simulink model "ep_DDMR_5Methods"  (Simulink 5.0)
settings: Solver=ode45  StartTime=0.0  StopTime=15  MaxStep=.1  MinStep=.001  RelTol=1e-3
values from neighbouring files (symbols this model uses):
  Gc = [2 2 3 4]    [init_ddmr.m]
  I_status = 0    [init_ddmr.m]
  IL_status = 1    [init_ddmr.m]
  PDIL_status = [1 2]    [init_ddmr.m]
libraries: dspsigattribs x15, dspmtrx3 x13, simulink x11, dspinverses x1
settings Model: LastModifiedBy=begawan  InitialStep=.001  MaxDataPoints=10000  BooleanDataType=off

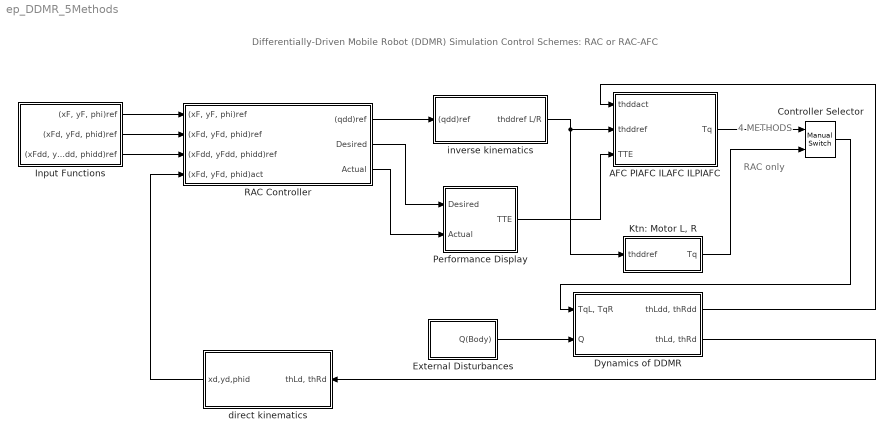
== system ep_DDMR_5Methods ==
  note: Differentially-Driven Mobile Robot (DDMR) Simulation
      | Control Schemes: RAC or RAC-AFC
  note: 4 METHODS
  note: RAC only
  "AFC PIAFC ILAFC ILPIAFC " : Subsystem  mask(6){GcAFC=on, GcPIAFC=off, GcILAFC=off, GcILPIAFC=off, pureIN=[2.4;2.4], PPhai=[0.2;0.2], DLa=[0.1;0.1], IN=[2.675;2.675], DIN=[0.71;0.71], Phai=[0.08;0.08], La=[0.06;0.06], Ktn=[0.0625;0.0625], Gear=[100;100]}
      mask prompts: GcAFC "Method: AFC"; GcPIAFC "Method: PIAFC"; GcILAFC "Method: ILAFC"; GcILPIAFC "Method: ILPIAFC"; pureIN "Pure IN"; PPhai "Proportional Phai (ILAFC)"; DLa "Derivative La (ILAFC)"; IN "Proportional IN"; DIN "Integral IN"; Phai "Proportional IL"; La "Integral IL"; Ktn "Motor Constant (Ktn)"; Gear "Motor's Gear Ratios"
      mask help: MM-RACAFC: Active Force Control Section
      mask CallbackString:
      | Gc = [1;1;1;2]
      | I_status = 0
      | IL_status = 0
      | PDIL_status = [3;4]
      | 
      | 
      | |Gc = [2;2;3;4]
      | I_status = 1
      | IL_status = 0
      | PDIL_status = [3;4]
      | 
      | 
      | |Gc = [1;1;1;2]
      | I_status = 0
      | IL_status = 1
      | PDIL_status = [1;2]
      | |Gc = [2;2;3;4]
      | I_status = 1
      | IL_status = 1
      | PDIL_status = [3;4]
      | |||||||||
  Controller Selector : simulink/Signal Routing/Manual Switch  sw=0  action=0
  Dynamics of DDMR : Subsystem  mask{phi=pi/2.4, d=0.3, r=0.11, mw=1, mc=40, b=.4, Ic=11.525, Im=0.05, Iw=0.05}
      mask prompts: phi "Vehicle initial orientation (phi)"; d "Distance between Po to Pc (d)"; r "Radius of Wheels (r)"; mw "Mass of wheel (mw)"; mc "Mass of platform (mc)"; b "(1/2)Width of vehicle (b)"; Ic "Inertia of platform about vertical axis (Ic)"; Im "Inertia of wheel about wheel diameter (Im)"; Iw "Inertia of wheel about wheel axis (Iw)"
  External Disturbances : Subsystem  mask(7){QstatusAFC=5, Qload=off, Qimpact=on, Qvibration=off, QQ=[5;5;20;-20]}
      mask prompts: QstatusAFC "Disturbance Status [1=enable 0=disable] or 0 to 1 as Gain"; Qload "Static (constant) Torques"; Qimpact "Impacts"; Qvibration "Vibration"; QQ "Constant Torques [L1 ; L2 ; Wheel_L ; Wheel_R] (Nm)"
      mask help: MM-RACAFC: Disturbances model
      mask init:
      | % Disturbance: Impact at t = x
      | Qpa1 = .9; Qpa2 = .9; QpaL = 5; QpaR = 5;
      | Qpf1 = 15; Qpf2 = 15; QpfL = 15; QpfR = 15;
      | Qpw1 = 2;  Qpw2 = 2;  QpwL = 2;  QpwR = 2;
      | Qpd1 = 8.5;  Qpd2 = 9.5;  QpdL = 10;  QpdR = 11;
      | 
      | % Disturbance: Vibration
      | Qsf1 = 20; Qsf2 = 18; QsfL = 14; QsfR = 14; %Hz
      | Qsa1 = .3; Qsa2 = .3; QsaL = 2;  QsaR = 2;  %N/m
      mask CallbackString:
      | |Qtype = [1;2;3;4];|Qtype = [5;6;7;8];
      | |Qtype = [9;10;11;12];
      | |
  Input Functions : Subsystem  mask{phiref=pi/2.4, InSet=4, Vcut=0.2, rinput=10}
      mask prompts: phiref "Vehicle Initial orientation (phiref)"; InSet "Input [ <1>Line-1 <2>Line-2 <3>Line-3 <4>Curve ]"; Vcut "Velocity of Running (Curve only)"; rinput "Radius of Curve"
  "Ktn: Motor L, R" : Subsystem  mask{Ktn=[0.0625;0.0625], Gear=[100;100]}
      mask prompts: Ktn "Motor Constant [L;R]"; Gear "Gear Ratios"
  Performance Display : Subsystem
  RAC Controller : Subsystem  mask{qinit=[10;0;pi/2.4], Kp=[450;450;.004], Kd=[320;320;.0017]}
      mask prompts: qinit "Vehicle initial position (xF, yF, phi) > (qinit)"; Kp "Proportional Constant (Kp)"; Kd "Differential Constant (Kd)"
  direct kinematics : Subsystem  Orientation=left  mask{phi=pi/2.4, b=0.4, r=0.11, lG=.3}
      mask prompts: phi "Vehicle initial orientation (phi)"; b "(1/2)Width of Body, b (m)"; r "Radius of wheels, r (m)"; lG "Distance between WG to WF (lG)"
  inverse kinematics : Subsystem  mask{phi=pi/2.4, b=0.4, r=0.11, lG=.3}
      mask prompts: phi "Vehicle initial orientation (phi)"; b "(1/2)Width of Body, b (m)"; r "Radius of wheels, r (m)"; lG "Distance between WG to WF (lG)"
  wires:
  Input Functions/2("(xFd, yFd, phid)ref") -> RAC Controller/2("(xFd, yFd, phid)ref")
  RAC Controller/1((qdd)ref) -> inverse kinematics/1((qdd)ref)
  Dynamics of DDMR/2("thLd, thRd") -> direct kinematics/1("thLd, thRd")
  Input Functions/1("(xF, yF, phi)ref") -> RAC Controller/1("(xF, yF, phi)ref")
  direct kinematics/1(xd,yd,phid) -> RAC Controller/4("(xFd, yFd, phid)act")
  Input Functions/3("(xFdd, yFdd, phidd)ref") -> RAC Controller/3("(xFdd, yFdd, phidd)ref")
  RAC Controller/3(Actual) -> Performance Display/2(Actual)
  RAC Controller/2(Desired) -> Performance Display/1(Desired)
  Dynamics of DDMR/1("thLdd, thRdd") -> "AFC PIAFC ILAFC ILPIAFC "/1(thddact)
  inverse kinematics/1(thddref L/R) -> "AFC PIAFC ILAFC ILPIAFC "/2(thddref), "Ktn: Motor L, R"/1(thddref)
  "AFC PIAFC ILAFC ILPIAFC "/1(Tq) -> Controller Selector/1
  Controller Selector/1 -> Dynamics of DDMR/1("TqL, TqR")
  "Ktn: Motor L, R"/1(Tq) -> Controller Selector/2
  External Disturbances/1(Q(Body)) -> Dynamics of DDMR/2(Q)
  Performance Display/1(TTE) -> "AFC PIAFC ILAFC ILPIAFC "/3(TTE)

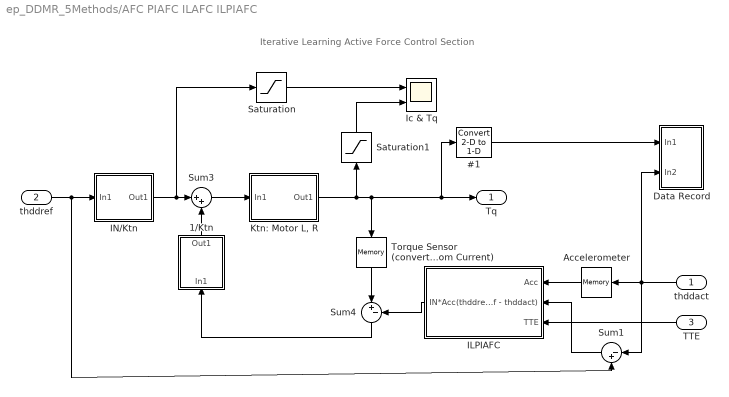
== system ep_DDMR_5Methods/AFC PIAFC ILAFC ILPIAFC  ==
  note: Iterative Learning Active Force Control Section
  thddact : Inport  Orientation=left
  thddref : Inport  Port=2
  TTE : Inport  Orientation=left  Port=3
  #1 : dspsigattribs/Convert 2-D to 1-D
  1/Ktn : Subsystem  Orientation=up
  Accelerometer : Memory  Orientation=left
  Data Record : Subsystem
  ILPIAFC : Subsystem  Orientation=left
  IN/Ktn : Subsystem
  Ic & Tq : Scope  NumInputPorts=2
      settings: TimeRange=7  YMin=-20~-200  YMax=60~200
  "Ktn: Motor L, R" : Subsystem
  Saturation : Saturate  UpperLimit=30  LowerLimit=-30
  Saturation1 : Saturate  Orientation=up  UpperLimit=30  LowerLimit=-30
  Sum1 : Sum  Orientation=left  Inputs=|-+  SaturateOnIntegerOverflow=on  InputSameDT=on
  Sum3 : Sum  Inputs=|++  SaturateOnIntegerOverflow=on  InputSameDT=on
  Sum4 : Sum  Orientation=down  Inputs=|+-  SaturateOnIntegerOverflow=on  InputSameDT=on
  Torque Sensor (converted from Current) : Memory  Orientation=down
  Tq : Outport
  wires:
  Sum3/1 -> "Ktn: Motor L, R"/1(In1)
  IN/Ktn/1(Out1) -> Sum3/1, Saturation/1
  ILPIAFC/1(IN*Acc) -> Sum4/2
  Sum4/1 -> 1/Ktn/1(In1)
  1/Ktn/1(Out1) -> Sum3/2
  thddref/1 -> IN/Ktn/1(In1), Sum1/2
  "Ktn: Motor L, R"/1(Out1) -> Torque Sensor (converted from Current)/1, Tq/1, #1/1, Saturation1/1
  Saturation/1 -> Ic & Tq/1
  Saturation1/1 -> Ic & Tq/2
  Accelerometer/1 -> ILPIAFC/1(Acc)
  Torque Sensor (converted from Current)/1 -> Sum4/1
  #1/1 -> Data Record/1(In1)
  Sum1/1 -> ILPIAFC/2((thddref - thddact))
  thddact/1 -> Accelerometer/1, Data Record/2(In2), Sum1/1
  TTE/1 -> ILPIAFC/3(TTE)

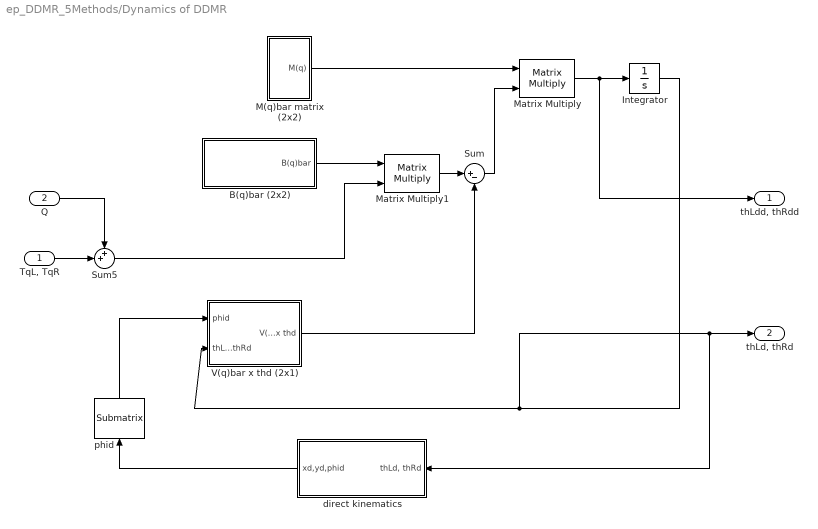
== system ep_DDMR_5Methods/Dynamics of DDMR ==
  "TqL, TqR" : Inport
  Q : Inport  Port=2
  B(q)bar (2x2) : Subsystem
  Integrator : Integrator
  M(q)bar matrix (2x2) : Subsystem
  Matrix Multiply : dspmtrx3/Matrix Multiply  numInputPorts=2  OptimizationLevel=None
  Matrix Multiply1 : dspmtrx3/Matrix Multiply  numInputPorts=2  OptimizationLevel=None
  Sum : Sum  Inputs=|+-  SaturateOnIntegerOverflow=on  InputSameDT=on
  Sum5 : Sum  Inputs=++|  SaturateOnIntegerOverflow=on  InputSameDT=on
  V(q)bar x thd (2x1) : Subsystem
  direct kinematics : Subsystem  Orientation=left
  phid : dspmtrx3/Submatrix  Orientation=up  RowSpan=Range of rows  RowStartMode=Index  RowStartIndex=3  RowEndMode=Last  RowEndIndex=1  ColSpan=Range of columns  ColStartMode=First  ColStartIndex=1  ColEndMode=Last  ColEndIndex=1
  "thLdd, thRdd" : Outport
  "thLd, thRd" : Outport  Port=2
  wires:
  M(q)bar matrix (2x2)/1(M(q)) -> Matrix Multiply/1
  B(q)bar (2x2)/1(B(q)bar) -> Matrix Multiply1/1
  Matrix Multiply1/1 -> Sum/1
  V(q)bar x thd (2x1)/1(V(q) bar x thd) -> Sum/2
  Sum/1 -> Matrix Multiply/2
  Matrix Multiply/1 -> Integrator/1, "thLdd, thRdd"/1
  Integrator/1 -> V(q)bar x thd (2x1)/2("thLd, thRd"), "thLd, thRd"/1, direct kinematics/1("thLd, thRd")
  direct kinematics/1(xd,yd,phid) -> phid/1
  phid/1 -> V(q)bar x thd (2x1)/1(phid)
  "TqL, TqR"/1 -> Sum5/2
  Sum5/1 -> Matrix Multiply1/2
  Q/1 -> Sum5/1

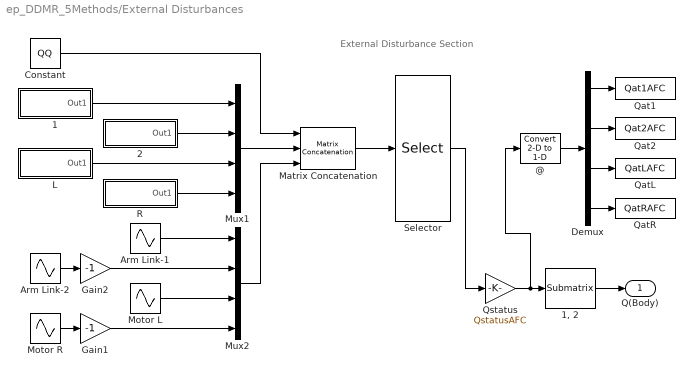
== system ep_DDMR_5Methods/External Disturbances ==
  note: External Disturbance Section
  1 : Subsystem
  "1, 2" : dspmtrx3/Submatrix  RowSpan=Range of rows  RowStartMode=Index  RowStartIndex=3  RowEndMode=Index  RowEndIndex=4  ColSpan=Range of columns  ColStartMode=First  ColStartIndex=1  ColEndMode=Last  ColEndIndex=1
  2 : Subsystem
  @ : dspsigattribs/Convert 2-D to 1-D
  Arm Link-1 : Sin  Amplitude=Qsa1  Frequency=Qsf1  SampleTime=0
  Arm Link-2 : Sin  Amplitude=Qsa2  Frequency=Qsf2  Phase=.5  SampleTime=0
  Constant : Constant  Value=QQ
  Demux : Demux
  Gain1 : Gain  Gain=-1  SaturateOnIntegerOverflow=on
  Gain2 : Gain  Gain=-1  SaturateOnIntegerOverflow=on
  L : Subsystem
  Matrix Concatenation : simulink/Math Operations/Matrix Concatenation  numInports=3  catMethod=Vertical
  Motor L : Sin  Amplitude=QsaL  Frequency=QsfL  SampleTime=0
  Motor R : Sin  Amplitude=QsaR  Frequency=QsfR  Phase=.5  SampleTime=0
  Mux1 : Mux
  Mux2 : Mux
  Qat1 : ToWorkspace  VariableName=Qat1AFC  SampleTime=-1  SaveFormat=Array
  Qat2 : ToWorkspace  VariableName=Qat2AFC  SampleTime=-1  SaveFormat=Array
  QatL : ToWorkspace  VariableName=QatLAFC  SampleTime=-1  SaveFormat=Array
  QatR : ToWorkspace  VariableName=QatRAFC  SampleTime=-1  SaveFormat=Array
  Qstatus : Gain  Gain=QstatusAFC  SaturateOnIntegerOverflow=on
  R : Subsystem
  Selector : Selector  Elements=Qtype  InputPortWidth=12
  Q(Body) : Outport
  wires:
  Selector/1 -> Qstatus/1
  Motor R/1 -> Gain1/1
  Constant/1 -> Matrix Concatenation/1
  Mux2/1 -> Matrix Concatenation/3
  Matrix Concatenation/1 -> Selector/1
  Arm Link-2/1 -> Gain2/1
  Motor L/1 -> Mux2/3
  Gain1/1 -> Mux2/4
  Gain2/1 -> Mux2/2
  Arm Link-1/1 -> Mux2/1
  R/1(Out1) -> Mux1/4
  2/1(Out1) -> Mux1/2
  Demux/1 -> Qat1/1
  Demux/2 -> Qat2/1
  Demux/3 -> QatL/1
  Demux/4 -> QatR/1
  1/1(Out1) -> Mux1/1
  Mux1/1 -> Matrix Concatenation/2
  L/1(Out1) -> Mux1/3
  @/1 -> Demux/1
  Qstatus/1 -> @/1, "1, 2"/1
  "1, 2"/1 -> Q(Body)/1

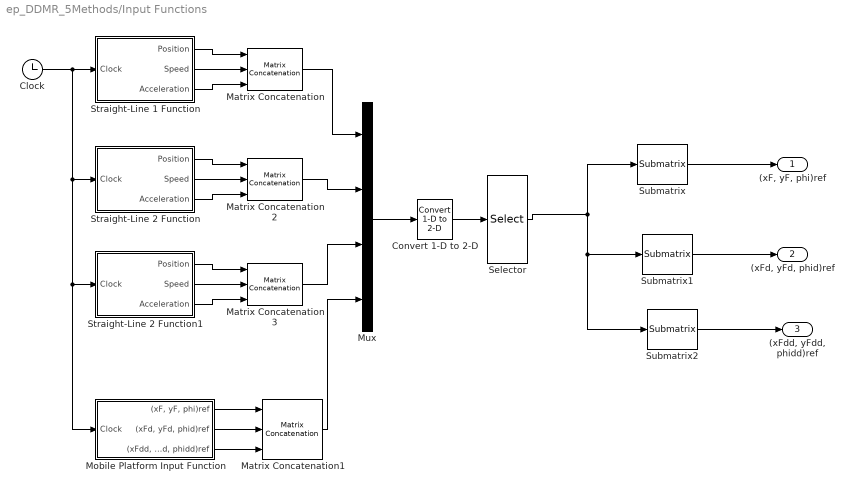
== system ep_DDMR_5Methods/Input Functions ==
  Clock : Clock
      settings: Decimation=10
  Convert 1-D to 2-D : dspsigattribs/Convert 1-D to 2-D  M=9  N=4  frameBasedOut=off
  Matrix Concatenation{,1..3} (4 alike) : simulink/Math Operations/Matrix Concatenation  numInports=3  catMethod=Vertical
  "Mobile Platform Input Function " : Subsystem
  Mux : Mux
  Selector : Selector  InputType=Matrix  ElementSrc=External  Elements=InSet  Rows=-1  Columns=InSet  InputPortWidth=2
  Straight-Line 1 Function : Subsystem
  Straight-Line 2 Function : Subsystem
  Straight-Line 2 Function1 : Subsystem
  Submatrix : dspmtrx3/Submatrix  RowSpan=Range of rows  RowStartMode=First  RowStartIndex=1  RowEndMode=Index  RowEndIndex=3  ColSpan=Range of columns  ColStartMode=First  ColStartIndex=1  ColEndMode=Last  ColEndIndex=1
  Submatrix1 : dspmtrx3/Submatrix  RowSpan=Range of rows  RowStartMode=Index  RowStartIndex=4  RowEndMode=Index  RowEndIndex=6  ColSpan=Range of columns  ColStartMode=First  ColStartIndex=1  ColEndMode=Last  ColEndIndex=1
  Submatrix2 : dspmtrx3/Submatrix  RowSpan=Range of rows  RowStartMode=Index  RowStartIndex=7  RowEndMode=Index  RowEndIndex=9  ColSpan=Range of columns  ColStartMode=First  ColStartIndex=1  ColEndMode=Last  ColEndIndex=1
  "(xF, yF, phi)ref" : Outport
  "(xFd, yFd, phid)ref" : Outport  Port=2
  "(xFdd, yFdd, phidd)ref" : Outport  Port=3
  wires:
  Clock/1 -> Straight-Line 1 Function/1(Clock), Straight-Line 2 Function/1(Clock), Straight-Line 2 Function1/1(Clock), "Mobile Platform Input Function "/1(Clock)
  Straight-Line 1 Function/1(Position) -> Matrix Concatenation/1
  Straight-Line 1 Function/2(Speed) -> Matrix Concatenation/2
  Straight-Line 1 Function/3(Acceleration) -> Matrix Concatenation/3
  "Mobile Platform Input Function "/1("(xF, yF, phi)ref") -> Matrix Concatenation1/1
  "Mobile Platform Input Function "/2("(xFd, yFd, phid)ref") -> Matrix Concatenation1/2
  "Mobile Platform Input Function "/3("(xFdd, yFdd, phidd)ref") -> Matrix Concatenation1/3
  Selector/1 -> Submatrix1/1, Submatrix2/1, Submatrix/1
  Matrix Concatenation/1 -> Mux/1
  Submatrix/1 -> "(xF, yF, phi)ref"/1
  Submatrix1/1 -> "(xFd, yFd, phid)ref"/1
  Submatrix2/1 -> "(xFdd, yFdd, phidd)ref"/1
  Mux/1 -> Convert 1-D to 2-D/1
  Convert 1-D to 2-D/1 -> Selector/1
  Straight-Line 2 Function/1(Position) -> Matrix Concatenation2/1
  Straight-Line 2 Function/2(Speed) -> Matrix Concatenation2/2
  Straight-Line 2 Function/3(Acceleration) -> Matrix Concatenation2/3
  Matrix Concatenation2/1 -> Mux/2
  Straight-Line 2 Function1/1(Position) -> Matrix Concatenation3/1
  Straight-Line 2 Function1/2(Speed) -> Matrix Concatenation3/2
  Straight-Line 2 Function1/3(Acceleration) -> Matrix Concatenation3/3
  Matrix Concatenation3/1 -> Mux/3
  Matrix Concatenation1/1 -> Mux/4

== system ep_DDMR_5Methods/Ktn: Motor L, R ==
  thddref : Inport
  Convert 2-D to 1-D : dspsigattribs/Convert 2-D to 1-D  Orientation=down
  Demux : Demux  Outputs=2
  Demux2 : Demux  Outputs=2
  IN/Ktn5 : Gain  Gain=Ktn(1)*Gear(1)  SaturateOnIntegerOverflow=on
  IN/Ktn6 : Gain  Gain=Ktn(2)*Gear(2)  SaturateOnIntegerOverflow=on
  Mux1 : Mux  Inputs=2
  To Workspace : ToWorkspace  VariableName=TqLpd1  SampleTime=-1  SaveFormat=Array
  To Workspace1 : ToWorkspace  VariableName=TqRpd1  SampleTime=-1  SaveFormat=Array
  Tq : Outport
  wires:
  Demux2/1 -> IN/Ktn5/1
  Demux2/2 -> IN/Ktn6/1
  IN/Ktn5/1 -> Mux1/1
  IN/Ktn6/1 -> Mux1/2
  thddref/1 -> Demux2/1
  Mux1/1 -> Tq/1, Convert 2-D to 1-D/1
  Convert 2-D to 1-D/1 -> Demux/1
  Demux/1 -> To Workspace/1
  Demux/2 -> To Workspace1/1

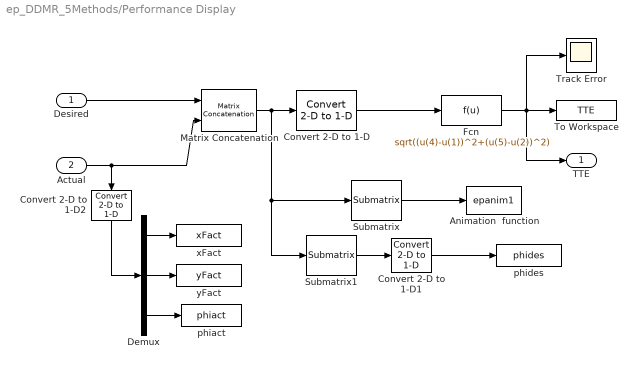
== system ep_DDMR_5Methods/Performance Display ==
  Desired : Inport
  Actual : Inport  Port=2
  Animation  function : S-Function  FunctionName=epanim1  Parameters=.4
      settings: DeleteFcn=if ~isempty(findobj('type','figure','name','onecart Animation'));close('onecart Animation'); end;
  Convert 2-D to 1-D : dspsigattribs/Convert 2-D to 1-D
  Convert 2-D to 1-D1 : dspsigattribs/Convert 2-D to 1-D
  Convert 2-D to 1-D2 : dspsigattribs/Convert 2-D to 1-D  Orientation=down
  Demux : Demux  Outputs=3
  Fcn : Fcn  Expr=sqrt((u(4)-u(1))^2+(u(5)-u(2))^2)
  Matrix Concatenation : simulink/Math Operations/Matrix Concatenation  numInports=2  catMethod=Vertical
  Submatrix : dspmtrx3/Submatrix  RowSpan=Range of rows  RowStartMode=Index  RowStartIndex=4  RowEndMode=Index  RowEndIndex=6  ColSpan=Range of columns  ColStartMode=First  ColStartIndex=1  ColEndMode=Last  ColEndIndex=1
  Submatrix1 : dspmtrx3/Submatrix  RowSpan=Range of rows  RowStartMode=Index  RowStartIndex=3  RowEndMode=Index  RowEndIndex=3  ColSpan=Range of columns  ColStartMode=First  ColStartIndex=1  ColEndMode=Last  ColEndIndex=1
  To Workspace : ToWorkspace  VariableName=TTE  SampleTime=-1  SaveFormat=Array
  Track Error : Scope
      settings: TickLabels=on  YMin=0  YMax=0.009  SaveName=ScopeData10
  phiact : ToWorkspace  VariableName=phiact  SampleTime=-1  SaveFormat=Array
  phides : ToWorkspace  VariableName=phides  SampleTime=-1  SaveFormat=Array
  xFact : ToWorkspace  VariableName=xFact  SampleTime=-1  SaveFormat=Array
  yFact : ToWorkspace  VariableName=yFact  SampleTime=-1  SaveFormat=Array
  TTE : Outport
  wires:
  Actual/1 -> Matrix Concatenation/2, Convert 2-D to 1-D2/1
  Matrix Concatenation/1 -> Convert 2-D to 1-D/1, Submatrix/1, Submatrix1/1
  Convert 2-D to 1-D/1 -> Fcn/1
  Desired/1 -> Matrix Concatenation/1
  Fcn/1 -> To Workspace/1, Track Error/1, TTE/1
  Submatrix/1 -> Animation  function/1
  Submatrix1/1 -> Convert 2-D to 1-D1/1
  Convert 2-D to 1-D1/1 -> phides/1
  Demux/1 -> xFact/1
  Demux/2 -> yFact/1
  Demux/3 -> phiact/1
  Convert 2-D to 1-D2/1 -> Demux/1

== system ep_DDMR_5Methods/RAC Controller ==
  "(xF, yF, phi)ref" : Inport
  "(xFd, yFd, phid)ref" : Inport  Port=2
  "(xFdd, yFdd, phidd)ref" : Inport  Port=3
  "(xFd, yFd, phid)act" : Inport  Port=4
  *Start of Position is HERE : Integrator  Orientation=up  InitialCondition=qinit
  "Kd " : Gain  Gain=Kd  SaturateOnIntegerOverflow=on
  Kp : Gain  Gain=Kp  SaturateOnIntegerOverflow=on
  Scope : Scope
      settings: SaveName=ScopeData2
  Sum : Sum  Inputs=+++  SaturateOnIntegerOverflow=on  InputSameDT=on
  Sum1 : Sum  Inputs=+-  SaturateOnIntegerOverflow=on  InputSameDT=on
  Sum2 : Sum  Inputs=+-  SaturateOnIntegerOverflow=on  InputSameDT=on
  (qdd)ref : Outport
  Desired : Outport  Orientation=left  Port=2
  Actual : Outport  Orientation=left  Port=3
  wires:
  Sum1/1 -> "Kd "/1
  Sum2/1 -> Kp/1
  "Kd "/1 -> Sum/2
  Kp/1 -> Sum/1, Scope/1
  *Start of Position is HERE/1 -> Sum2/2, Actual/1
  "(xF, yF, phi)ref"/1 -> Sum2/1, Desired/1
  Sum/1 -> (qdd)ref/1
  "(xFd, yFd, phid)ref"/1 -> Sum1/1
  "(xFd, yFd, phid)act"/1 -> *Start of Position is HERE/1, Sum1/2
  "(xFdd, yFdd, phidd)ref"/1 -> Sum/3

== system ep_DDMR_5Methods/direct kinematics ==
  "thLd, thRd" : Inport
  Integrator : Integrator  Orientation=left  InitialCondition=phi
  Matrix Multiply : dspmtrx3/Matrix Multiply  numInputPorts=2  OptimizationLevel=None
  S(q) matrix (3x2)1 : Subsystem
  xd,yd,phid : Outport
  wires:
  "thLd, thRd"/1 -> Matrix Multiply/2
  Matrix Multiply/1 -> xd,yd,phid/1, Integrator/1
  Integrator/1 -> S(q) matrix (3x2)1/1(phi)
  S(q) matrix (3x2)1/1(S(q)) -> Matrix Multiply/1

== system ep_DDMR_5Methods/inverse kinematics ==
  (qdd)ref : Inport
  Convert 1-D to 2-D : dspsigattribs/Convert 1-D to 2-D  M=3  N=1  frameBasedOut=off
  Integrator : Integrator  Orientation=up  InitialCondition=phi
  Matrix Multiply : dspmtrx3/Matrix Multiply  numInputPorts=2  OptimizationLevel=None
  Pseudoinverse : dspinverses/Pseudoinverse
  S(q) matrix (3x2)1 : Subsystem
  thddref L/R : Outport
  wires:
  Pseudoinverse/1 -> Matrix Multiply/1
  (qdd)ref/1 -> Convert 1-D to 2-D/1, Integrator/1
  Matrix Multiply/1 -> thddref L/R/1
  Convert 1-D to 2-D/1 -> Matrix Multiply/2
  Integrator/1 -> S(q) matrix (3x2)1/1(phi)
  S(q) matrix (3x2)1/1(S(q)) -> Pseudoinverse/1

== system ep_DDMR_5Methods/AFC PIAFC ILAFC ILPIAFC /1/Ktn ==
  In1 : Inport
  Demux4 : Demux  Outputs=2
  IN/Ktn10 : Gain  Gain=1/(Ktn(2)*Gear(2))  SaturateOnIntegerOverflow=on
  IN/Ktn9 : Gain  Gain=1/(Ktn(1)*Gear(1))  SaturateOnIntegerOverflow=on
  Mux2 : Mux  Inputs=2
  Out1 : Outport
  wires:
  Demux4/1 -> IN/Ktn9/1
  Demux4/2 -> IN/Ktn10/1
  IN/Ktn9/1 -> Mux2/1
  IN/Ktn10/1 -> Mux2/2
  In1/1 -> Demux4/1
  Mux2/1 -> Out1/1

== system ep_DDMR_5Methods/AFC PIAFC ILAFC ILPIAFC /Data Record ==
  In1 : Inport
  In2 : Inport  Orientation=up  Port=2
  # : dspsigattribs/Convert 2-D to 1-D  Orientation=up
  Demux : Demux  Outputs=2
  Demux1 : Demux  Outputs=2
  TqL : ToWorkspace  VariableName=TqLPIAFC  SampleTime=-1  SaveFormat=Array
  TqR : ToWorkspace  VariableName=TqRPIAFC  SampleTime=-1  SaveFormat=Array
  thLdd : ToWorkspace  VariableName=thLddPIAFC  SampleTime=-1  SaveFormat=Array
  thRdd : ToWorkspace  VariableName=thRddPIAFC  SampleTime=-1  SaveFormat=Array
  wires:
  #/1 -> Demux1/1
  In2/1 -> #/1
  In1/1 -> Demux/1
  Demux/1 -> TqL/1
  Demux/2 -> TqR/1
  Demux1/1 -> thLdd/1
  Demux1/2 -> thRdd/1

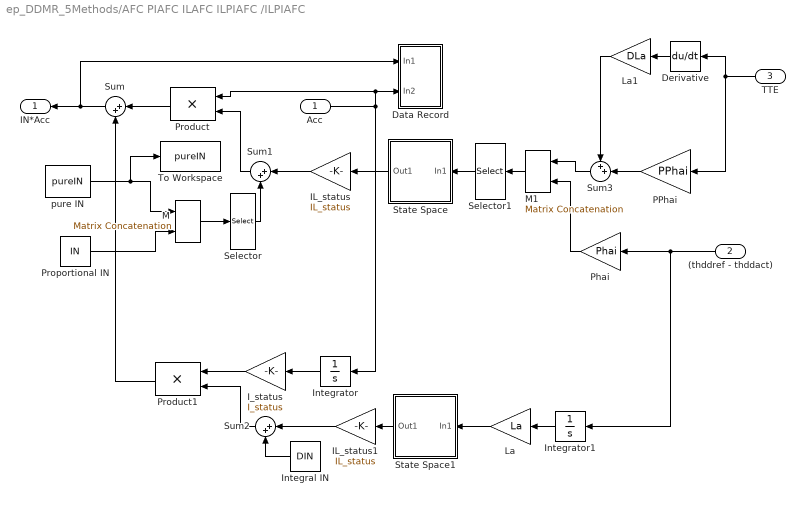
== system ep_DDMR_5Methods/AFC PIAFC ILAFC ILPIAFC /ILPIAFC ==
  Acc : Inport
  (thddref - thddact) : Inport  Orientation=left  Port=2
  TTE : Inport  Orientation=left  Port=3
  Data Record : Subsystem
  Derivative : Derivative  Orientation=left
  IL_status : Gain  Orientation=left  Gain=IL_status  SaturateOnIntegerOverflow=on
  IL_status1 : Gain  Orientation=left  Gain=IL_status  SaturateOnIntegerOverflow=on
  I_status : Gain  Orientation=left  Gain=I_status  SaturateOnIntegerOverflow=on
  Integral IN : Constant  Orientation=left  Value=DIN
  Integrator : Integrator  Orientation=left
  Integrator1 : Integrator  Orientation=left
  La : Gain  Orientation=left  Gain=La  SaturateOnIntegerOverflow=on
  La1 : Gain  Orientation=left  Gain=DLa  SaturateOnIntegerOverflow=on
  M : simulink/Math Operations/Matrix Concatenation  numInports=2  catMethod=Vertical
  M1 : simulink/Math Operations/Matrix Concatenation  Orientation=left  numInports=2  catMethod=Vertical
  PPhai : Gain  Orientation=left  Gain=PPhai  SaturateOnIntegerOverflow=on
  Phai : Gain  Orientation=left  Gain=Phai  SaturateOnIntegerOverflow=on
  Product : Product  Orientation=left  SaturateOnIntegerOverflow=on
  Product1 : Product  Orientation=left  SaturateOnIntegerOverflow=on
  "Proportional IN " : Constant  Value=IN
  Selector : Selector  Elements=[Gc(3);Gc(4)]  InputPortWidth=4
  Selector1 : Selector  Orientation=left  Elements=[PDIL_status(1);PDIL_status(2)]  InputPortWidth=4
  State Space : Subsystem  Orientation=left
  State Space1 : Subsystem  Orientation=left
  Sum : Sum  Orientation=left  Inputs=|++  SaturateOnIntegerOverflow=on
  Sum1 : Sum  Orientation=left  Inputs=|++  SaturateOnIntegerOverflow=on
  Sum2 : Sum  Orientation=left  Inputs=|++  SaturateOnIntegerOverflow=on
  Sum3 : Sum  Orientation=left  Inputs=++|  SaturateOnIntegerOverflow=on
  To Workspace : ToWorkspace  VariableName=pureIN  SampleTime=-1  SaveFormat=Array
  pure IN : Constant  Value=pureIN
  IN*Acc : Outport  Orientation=left
  wires:
  Acc/1 -> Data Record/2(In2), Integrator/1, Product/1
  Product/1 -> Sum/1
  Product1/1 -> Sum/2
  Sum/1 -> IN*Acc/1, Data Record/1(In1)
  Sum1/1 -> Product/2
  Sum2/1 -> Product1/2
  Integral IN/1 -> Sum2/2
  State Space/1(Out1) -> IL_status/1
  State Space1/1(Out1) -> IL_status1/1
  La/1 -> State Space1/1(In1)
  Integrator1/1 -> La/1
  (thddref - thddact)/1 -> Integrator1/1, Phai/1
  IL_status/1 -> Sum1/1
  IL_status1/1 -> Sum2/1
  I_status/1 -> Product1/1
  Integrator/1 -> I_status/1
  M/1 -> Selector/1
  Selector/1 -> Sum1/2
  pure IN/1 -> M/1, To Workspace/1
  "Proportional IN "/1 -> M/2
  La1/1 -> Sum3/1
  Derivative/1 -> La1/1
  PPhai/1 -> Sum3/2
  TTE/1 -> PPhai/1, Derivative/1
  Selector1/1 -> State Space/1(In1)
  Sum3/1 -> M1/1
  Phai/1 -> M1/2
  M1/1 -> Selector1/1

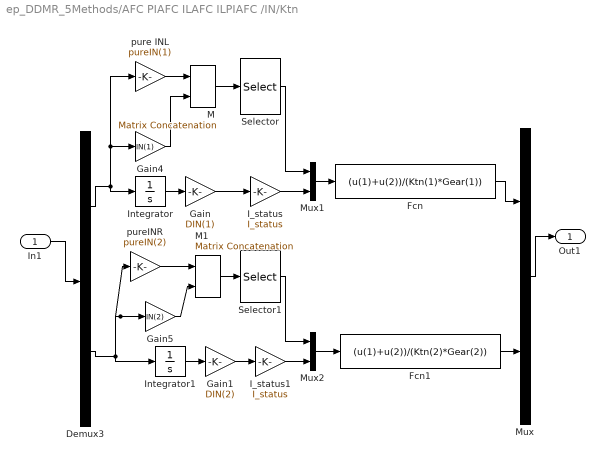
== system ep_DDMR_5Methods/AFC PIAFC ILAFC ILPIAFC /IN/Ktn ==
  In1 : Inport
  Demux3 : Demux  Outputs=2
  Fcn : Fcn  Expr=(u(1)+u(2))/(Ktn(1)*Gear(1))
  Fcn1 : Fcn  Expr=(u(1)+u(2))/(Ktn(2)*Gear(2))
  Gain : Gain  Gain=DIN(1)  SaturateOnIntegerOverflow=on
  Gain1 : Gain  Gain=DIN(2)  SaturateOnIntegerOverflow=on
  Gain4 : Gain  Gain=IN(1)  SaturateOnIntegerOverflow=on
  Gain5 : Gain  Gain=IN(2)  SaturateOnIntegerOverflow=on
  I_status : Gain  Gain=I_status  SaturateOnIntegerOverflow=on
  I_status1 : Gain  Gain=I_status  SaturateOnIntegerOverflow=on
  Integrator : Integrator
  Integrator1 : Integrator
  M : simulink/Math Operations/Matrix Concatenation  numInports=2  catMethod=Vertical
  M1 : simulink/Math Operations/Matrix Concatenation  numInports=2  catMethod=Vertical
  Mux : Mux  Inputs=2
  Mux1 : Mux  Inputs=2
  Mux2 : Mux  Inputs=2
  Selector : Selector  Elements=Gc(1)  InputPortWidth=2
  Selector1 : Selector  Elements=Gc(2)  InputPortWidth=2
  pure INL : Gain  Gain=pureIN(1)  SaturateOnIntegerOverflow=on
  pureINR : Gain  Gain=pureIN(2)  SaturateOnIntegerOverflow=on
  Out1 : Outport
  wires:
  Fcn/1 -> Mux/1
  In1/1 -> Demux3/1
  Mux/1 -> Out1/1
  Mux1/1 -> Fcn/1
  Mux2/1 -> Fcn1/1
  Gain/1 -> I_status/1
  Gain1/1 -> I_status1/1
  Fcn1/1 -> Mux/2
  Demux3/1 -> Integrator/1, Gain4/1, pure INL/1
  Demux3/2 -> Integrator1/1, Gain5/1, pureINR/1
  I_status/1 -> Mux1/2
  I_status1/1 -> Mux2/2
  Integrator1/1 -> Gain1/1
  Integrator/1 -> Gain/1
  Selector/1 -> Mux1/1
  Gain4/1 -> M/2
  pure INL/1 -> M/1
  M/1 -> Selector/1
  M1/1 -> Selector1/1
  Gain5/1 -> M1/2
  pureINR/1 -> M1/1
  Selector1/1 -> Mux2/1

== system ep_DDMR_5Methods/AFC PIAFC ILAFC ILPIAFC /Ktn: Motor L, R ==
  In1 : Inport
  Demux2 : Demux  Outputs=2
  IN/Ktn5 : Gain  Gain=Ktn(1)*Gear(1)  SaturateOnIntegerOverflow=on
  IN/Ktn6 : Gain  Gain=Ktn(2)*Gear(2)  SaturateOnIntegerOverflow=on
  Mux1 : Mux  Inputs=2
  Out1 : Outport
  wires:
  Demux2/1 -> IN/Ktn5/1
  Demux2/2 -> IN/Ktn6/1
  IN/Ktn5/1 -> Mux1/1
  IN/Ktn6/1 -> Mux1/2
  In1/1 -> Demux2/1
  Mux1/1 -> Out1/1

== system ep_DDMR_5Methods/Dynamics of DDMR/B(q)bar (2x2) ==
  Constant1 : Constant  Value=0
  Constant2 : Constant
  Constant3 : Constant  Value=0
  Constant4 : Constant
  Convert 1-D to 2-D : dspsigattribs/Convert 1-D to 2-D  M=2  N=2  frameBasedOut=off
  Mux : Mux
  B(q)bar : Outport
  wires:
  Mux/1 -> Convert 1-D to 2-D/1
  Constant2/1 -> Mux/1
  Constant1/1 -> Mux/2
  Constant3/1 -> Mux/3
  Constant4/1 -> Mux/4
  Convert 1-D to 2-D/1 -> B(q)bar/1

== system ep_DDMR_5Methods/Dynamics of DDMR/M(q)bar matrix (2x2) ==
  Convert 1-D to 2-D : dspsigattribs/Convert 1-D to 2-D  M=2  N=2  frameBasedOut=off
  M11 : Constant  Value=(r^2)/(4*(b^2))*((mc+2*mw)*(b^2)+(mc*(d^2)+2*mw*(b^2)+Ic+2*Im))+Iw
  M12 : Constant  Value=(r^2)/(4*(b^2))*((mc+2*mw)*(b^2)-(mc*(d^2)+2*mw*(b^2)+Ic+2*Im))
  M21 : Constant  Value=(r^2)/(4*(b^2))*((mc+2*mw)*(b^2)-(mc*(d^2)+2*mw*(b^2)+Ic+2*Im))
  M22 : Constant  Value=(r^2)/(4*(b^2))*((mc+2*mw)*(b^2)+(mc*(d^2)+2*mw*(b^2)+Ic+2*Im))+Iw
  Mux : Mux
  M(q) : Outport
  wires:
  M11/1 -> Mux/1
  M12/1 -> Mux/2
  M21/1 -> Mux/3
  M22/1 -> Mux/4
  Mux/1 -> Convert 1-D to 2-D/1
  Convert 1-D to 2-D/1 -> M(q)/1

== system ep_DDMR_5Methods/Dynamics of DDMR/V(q)bar x thd (2x1) ==
  phid : Inport
  "thLd, thRd" : Inport  Port=2
  Matrix Multiply3 : dspmtrx3/Matrix Multiply  numInputPorts=2  OptimizationLevel=None
  V(q,qd)bar (3x1) : Subsystem
  V(q) bar x thd : Outport
  wires:
  Matrix Multiply3/1 -> V(q) bar x thd/1
  V(q,qd)bar (3x1)/1(V(q,qd)bar) -> Matrix Multiply3/1
  phid/1 -> V(q,qd)bar (3x1)/1(phid)
  "thLd, thRd"/1 -> Matrix Multiply3/2

== system ep_DDMR_5Methods/Dynamics of DDMR/direct kinematics ==
  "thLd, thRd" : Inport
  Integrator : Integrator  Orientation=left  InitialCondition=phi
  Matrix Multiply : dspmtrx3/Matrix Multiply  numInputPorts=2  OptimizationLevel=None
  S(q) matrix (3x2)1 : Subsystem
  xd,yd,phid : Outport
  wires:
  "thLd, thRd"/1 -> Matrix Multiply/2
  Matrix Multiply/1 -> xd,yd,phid/1, Integrator/1
  Integrator/1 -> S(q) matrix (3x2)1/1(phi)
  S(q) matrix (3x2)1/1(S(q)) -> Matrix Multiply/1

== system ep_DDMR_5Methods/External Disturbances/1 ==
  PG1d : DiscretePulseGenerator  PulseType=Time based  Amplitude=-Qpa1/2  Period=Qpf1  PulseWidth=Qpw1  PhaseDelay=Qpd1+.3
  PG1u : DiscretePulseGenerator  PulseType=Time based  Amplitude=Qpa1  Period=Qpf1  PulseWidth=Qpw1  PhaseDelay=Qpd1
  Sum : Sum  Inputs=|++  SaturateOnIntegerOverflow=on
  Out1 : Outport
  wires:
  PG1d/1 -> Sum/2
  PG1u/1 -> Sum/1
  Sum/1 -> Out1/1

== system ep_DDMR_5Methods/External Disturbances/2 ==
  PG1d : DiscretePulseGenerator  PulseType=Time based  Amplitude=-Qpa2/2  Period=Qpf2  PulseWidth=Qpw2  PhaseDelay=Qpd2+.3
  PG1u : DiscretePulseGenerator  PulseType=Time based  Amplitude=Qpa2  Period=Qpf2  PulseWidth=Qpw2  PhaseDelay=Qpd2
  Sum : Sum  Inputs=|++  SaturateOnIntegerOverflow=on
  Out1 : Outport
  wires:
  PG1d/1 -> Sum/2
  PG1u/1 -> Sum/1
  Sum/1 -> Out1/1

== system ep_DDMR_5Methods/External Disturbances/L ==
  PG1d : DiscretePulseGenerator  PulseType=Time based  Amplitude=-QpaL/2  Period=QpfL  PulseWidth=QpwL  PhaseDelay=QpdL+.3
  PG1u : DiscretePulseGenerator  PulseType=Time based  Amplitude=QpaL  Period=QpfL  PulseWidth=QpwL  PhaseDelay=QpdL
  Sum : Sum  Inputs=|++  SaturateOnIntegerOverflow=on
  Out1 : Outport
  wires:
  PG1d/1 -> Sum/2
  PG1u/1 -> Sum/1
  Sum/1 -> Out1/1

== system ep_DDMR_5Methods/External Disturbances/R ==
  PG1d : DiscretePulseGenerator  PulseType=Time based  Amplitude=-QpaR/2  Period=QpfR  PulseWidth=QpwR  PhaseDelay=QpdR+.3
  PG1u : DiscretePulseGenerator  PulseType=Time based  Amplitude=QpaR  Period=QpfR  PulseWidth=QpwR  PhaseDelay=QpdR
  Sum : Sum  Inputs=|++  SaturateOnIntegerOverflow=on
  Out1 : Outport
  wires:
  PG1d/1 -> Sum/2
  PG1u/1 -> Sum/1
  Sum/1 -> Out1/1

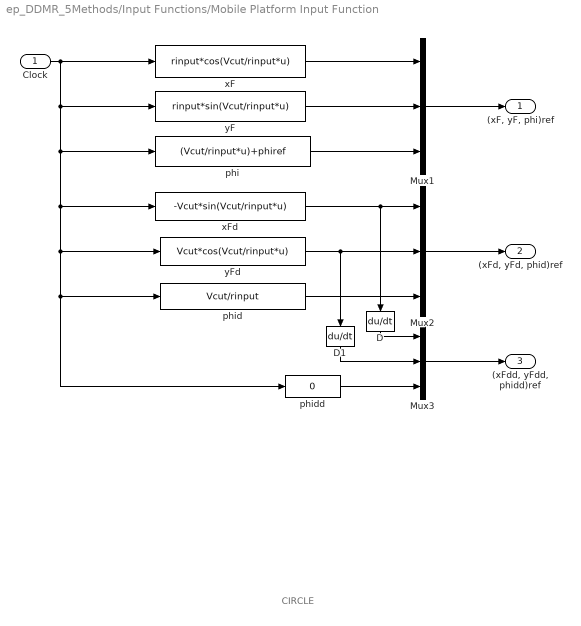
== system ep_DDMR_5Methods/Input Functions/Mobile Platform Input Function  ==
  note: CIRCLE
  Clock : Inport
  D : Derivative  Orientation=down
  D1 : Derivative  Orientation=down
  Mux1 : Mux  Inputs=3
  Mux2 : Mux  Inputs=3
  Mux3 : Mux  Inputs=3
  phi : Fcn  Expr=(Vcut/rinput*u)+phiref
  phid : Fcn  Expr=Vcut/rinput
  phidd : Fcn  Expr=0
  xF : Fcn  Expr=rinput*cos(Vcut/rinput*u)
  xFd : Fcn  Expr=-Vcut*sin(Vcut/rinput*u)
  yF : Fcn  Expr=rinput*sin(Vcut/rinput*u)
  yFd : Fcn  Expr=Vcut*cos(Vcut/rinput*u)
  "(xF, yF, phi)ref" : Outport
  "(xFd, yFd, phid)ref" : Outport  Port=2
  "(xFdd, yFdd, phidd)ref" : Outport  Port=3
  wires:
  yF/1 -> Mux1/2
  yFd/1 -> Mux2/2, D1/1
  xFd/1 -> Mux2/1, D/1
  xF/1 -> Mux1/1
  phi/1 -> Mux1/3
  phid/1 -> Mux2/3
  phidd/1 -> Mux3/3
  Mux1/1 -> "(xF, yF, phi)ref"/1
  Mux2/1 -> "(xFd, yFd, phid)ref"/1
  Mux3/1 -> "(xFdd, yFdd, phidd)ref"/1
  Clock/1 -> xF/1, phid/1, phidd/1, yFd/1, xFd/1, phi/1, yF/1
  D/1 -> Mux3/1
  D1/1 -> Mux3/2

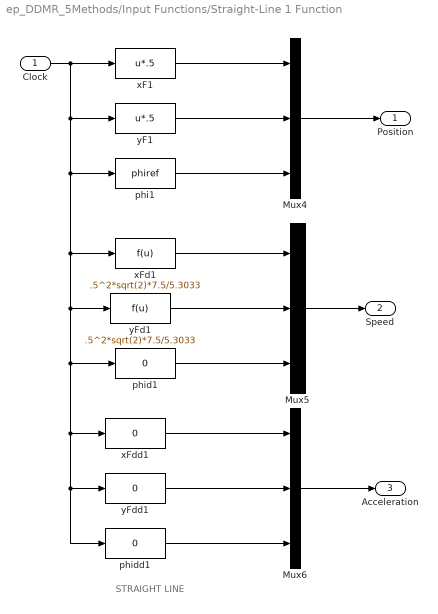
== system ep_DDMR_5Methods/Input Functions/Straight-Line 1 Function ==
  note: STRAIGHT LINE
  Clock : Inport
  Mux4 : Mux  Inputs=3
  Mux5 : Mux  Inputs=3
  Mux6 : Mux  Inputs=3
  phi1 : Fcn  Expr=phiref
  phid1 : Fcn  Expr=0
  phidd1 : Fcn  Expr=0
  xF1 : Fcn  Expr=u*.5
  xFd1 : Fcn  Expr=.5^2*sqrt(2)*7.5/5.3033
  xFdd1 : Fcn  Expr=0
  yF1 : Fcn  Expr=u*.5
  yFd1 : Fcn  Expr=.5^2*sqrt(2)*7.5/5.3033
  yFdd1 : Fcn  Expr=0
  Position : Outport
  Speed : Outport  Port=2
  Acceleration : Outport  Port=3
  wires:
  Clock/1 -> xF1/1, phi1/1, yFd1/1, phidd1/1, yFdd1/1, xFdd1/1, phid1/1, xFd1/1, yF1/1
  Mux4/1 -> Position/1
  Mux5/1 -> Speed/1
  Mux6/1 -> Acceleration/1
  xF1/1 -> Mux4/1
  phi1/1 -> Mux4/3
  yFd1/1 -> Mux5/2
  phid1/1 -> Mux5/3
  xFdd1/1 -> Mux6/1
  yFdd1/1 -> Mux6/2
  phidd1/1 -> Mux6/3
  yF1/1 -> Mux4/2
  xFd1/1 -> Mux5/1

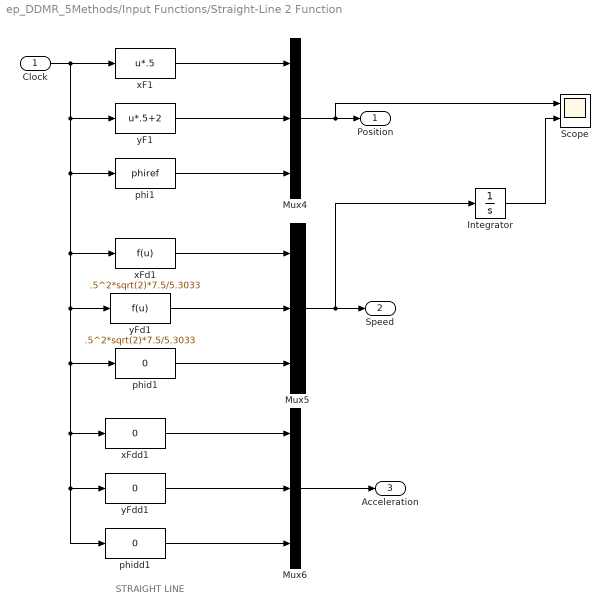
== system ep_DDMR_5Methods/Input Functions/Straight-Line 2 Function ==
  note: STRAIGHT LINE
  Clock : Inport
  Integrator : Integrator  InitialCondition=[-2;2;pi/4]
  Mux4 : Mux  Inputs=3
  Mux5 : Mux  Inputs=3
  Mux6 : Mux  Inputs=3
  Scope : Scope  NumInputPorts=2
      settings: YMin=-5~-5  YMax=5~5
  phi1 : Fcn  Expr=phiref
  phid1 : Fcn  Expr=0
  phidd1 : Fcn  Expr=0
  xF1 : Fcn  Expr=u*.5
  xFd1 : Fcn  Expr=.5^2*sqrt(2)*7.5/5.3033
  xFdd1 : Fcn  Expr=0
  yF1 : Fcn  Expr=u*.5+2
  yFd1 : Fcn  Expr=.5^2*sqrt(2)*7.5/5.3033
  yFdd1 : Fcn  Expr=0
  Position : Outport
  Speed : Outport  Port=2
  Acceleration : Outport  Port=3
  wires:
  Clock/1 -> xF1/1, phi1/1, yFd1/1, phidd1/1, yFdd1/1, xFdd1/1, phid1/1, xFd1/1, yF1/1
  Mux4/1 -> Position/1, Scope/1
  Mux5/1 -> Speed/1, Integrator/1
  Mux6/1 -> Acceleration/1
  xF1/1 -> Mux4/1
  phi1/1 -> Mux4/3
  yFd1/1 -> Mux5/2
  phid1/1 -> Mux5/3
  xFdd1/1 -> Mux6/1
  yFdd1/1 -> Mux6/2
  phidd1/1 -> Mux6/3
  yF1/1 -> Mux4/2
  xFd1/1 -> Mux5/1
  Integrator/1 -> Scope/2

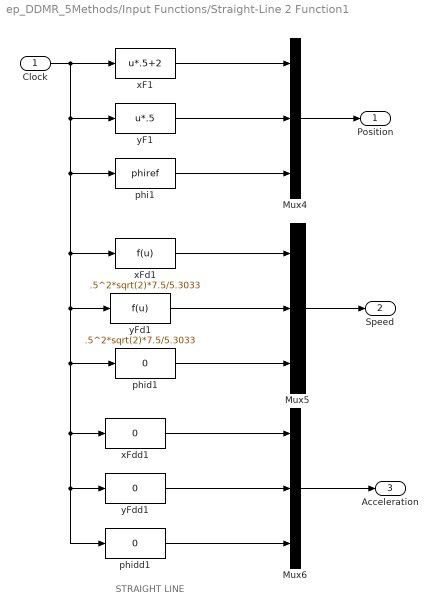
== system ep_DDMR_5Methods/Input Functions/Straight-Line 2 Function1 ==
  note: STRAIGHT LINE
  Clock : Inport
  Mux4 : Mux  Inputs=3
  Mux5 : Mux  Inputs=3
  Mux6 : Mux  Inputs=3
  phi1 : Fcn  Expr=phiref
  phid1 : Fcn  Expr=0
  phidd1 : Fcn  Expr=0
  xF1 : Fcn  Expr=u*.5+2
  xFd1 : Fcn  Expr=.5^2*sqrt(2)*7.5/5.3033
  xFdd1 : Fcn  Expr=0
  yF1 : Fcn  Expr=u*.5
  yFd1 : Fcn  Expr=.5^2*sqrt(2)*7.5/5.3033
  yFdd1 : Fcn  Expr=0
  Position : Outport
  Speed : Outport  Port=2
  Acceleration : Outport  Port=3
  wires:
  Clock/1 -> xF1/1, phi1/1, yFd1/1, phidd1/1, yFdd1/1, xFdd1/1, phid1/1, xFd1/1, yF1/1
  Mux4/1 -> Position/1
  Mux5/1 -> Speed/1
  Mux6/1 -> Acceleration/1
  xF1/1 -> Mux4/1
  phi1/1 -> Mux4/3
  yFd1/1 -> Mux5/2
  phid1/1 -> Mux5/3
  xFdd1/1 -> Mux6/1
  yFdd1/1 -> Mux6/2
  phidd1/1 -> Mux6/3
  yF1/1 -> Mux4/2
  xFd1/1 -> Mux5/1

== system ep_DDMR_5Methods/direct kinematics/S(q) matrix (3x2)1 ==
  phi : Inport
  Constant1 : Constant  Value=r/(2*b)
  Constant2 : Constant  Value=-r/(2*b)
  Convert 1-D to 2-D : dspsigattribs/Convert 1-D to 2-D  M=3  N=2  frameBasedOut=off
  Fcn : Fcn  Expr=r/2*cos(u(3))+lG*r/(2*b)*sin(u(3))
  Fcn1 : Fcn  Expr=r/2*sin(u(3))-lG*r/(2*b)*cos(u(3))
  Fcn2 : Fcn  Expr=r/2*cos(u(3))-lG*r/(2*b)*sin(u(3))
  Fcn3 : Fcn  Expr=r/2*sin(u(3))+lG*r/(2*b)*cos(u(3))
  Mux : Mux  Inputs=6
  S(q) : Outport
  wires:
  Mux/1 -> Convert 1-D to 2-D/1
  Convert 1-D to 2-D/1 -> S(q)/1
  phi/1 -> Fcn3/1, Fcn2/1, Fcn/1, Fcn1/1
  Fcn/1 -> Mux/1
  Fcn1/1 -> Mux/2
  Constant2/1 -> Mux/3
  Fcn2/1 -> Mux/4
  Fcn3/1 -> Mux/5
  Constant1/1 -> Mux/6

== system ep_DDMR_5Methods/inverse kinematics/S(q) matrix (3x2)1 ==
  phi : Inport
  Constant1 : Constant  Value=r/(2*b)
  Constant2 : Constant  Value=-r/(2*b)
  Convert 1-D to 2-D : dspsigattribs/Convert 1-D to 2-D  M=3  N=2  frameBasedOut=off
  Fcn : Fcn  Expr=r/2*cos(u(3))+lG*r/(2*b)*sin(u(3))
  Fcn1 : Fcn  Expr=r/2*sin(u(3))-lG*r/(2*b)*cos(u(3))
  Fcn2 : Fcn  Expr=r/2*cos(u(3))-lG*r/(2*b)*sin(u(3))
  Fcn3 : Fcn  Expr=r/2*sin(u(3))+lG*r/(2*b)*cos(u(3))
  Mux : Mux  Inputs=6
  S(q) : Outport
  wires:
  Mux/1 -> Convert 1-D to 2-D/1
  Convert 1-D to 2-D/1 -> S(q)/1
  phi/1 -> Fcn3/1, Fcn2/1, Fcn/1, Fcn1/1
  Fcn/1 -> Mux/1
  Fcn1/1 -> Mux/2
  Constant2/1 -> Mux/3
  Fcn2/1 -> Mux/4
  Fcn3/1 -> Mux/5
  Constant1/1 -> Mux/6

== system ep_DDMR_5Methods/AFC PIAFC ILAFC ILPIAFC /ILPIAFC/Data Record ==
  In1 : Inport
  In2 : Inport  Port=2
  Demux1 : Demux  Outputs=2
  Demux2 : Demux  Outputs=2
  Fcn : Fcn  Expr=u(2)/u(1)
  Fcn1 : Fcn  Expr=u(2)/u(1)
  Memory : Memory
  Mux : Mux  Inputs=2
  Mux1 : Mux  Inputs=2
  To Workspace2 : ToWorkspace  VariableName=INLPIAFC  SampleTime=-1  SaveFormat=Array
  To Workspace3 : ToWorkspace  VariableName=INRPIAFC  SampleTime=-1  SaveFormat=Array
  wires:
  Mux/1 -> Fcn/1
  Mux1/1 -> Fcn1/1
  Fcn/1 -> To Workspace2/1
  Fcn1/1 -> To Workspace3/1
  Demux1/1 -> Mux/1
  Demux1/2 -> Mux1/1
  Demux2/1 -> Mux/2
  Demux2/2 -> Mux1/2
  Memory/1 -> Demux2/1
  In1/1 -> Demux1/1
  In2/1 -> Memory/1

== system ep_DDMR_5Methods/AFC PIAFC ILAFC ILPIAFC /ILPIAFC/State Space ==
  In1 : Inport  Orientation=left
  Demux : Demux  Orientation=left  Outputs=2
  Mux : Mux  Orientation=left  Inputs=2
  State-Space4 : StateSpace  Orientation=left  A=0.05  B=0.2  D=0
  State-Space5 : StateSpace  Orientation=left  A=0.05  B=0.2  D=0
  Out1 : Outport  Orientation=left
  wires:
  Demux/1 -> State-Space5/1
  Demux/2 -> State-Space4/1
  State-Space5/1 -> Mux/1
  State-Space4/1 -> Mux/2
  In1/1 -> Demux/1
  Mux/1 -> Out1/1

== system ep_DDMR_5Methods/AFC PIAFC ILAFC ILPIAFC /ILPIAFC/State Space1 ==
  In1 : Inport  Orientation=left
  Demux : Demux  Orientation=left  Outputs=2
  Mux : Mux  Orientation=left  Inputs=2
  State-Space4 : StateSpace  Orientation=left  A=0.05  B=0.2  D=0
  State-Space5 : StateSpace  Orientation=left  A=0.05  B=0.2  D=0
  Out1 : Outport  Orientation=left
  wires:
  Demux/1 -> State-Space5/1
  Demux/2 -> State-Space4/1
  State-Space5/1 -> Mux/1
  State-Space4/1 -> Mux/2
  In1/1 -> Demux/1
  Mux/1 -> Out1/1

== system ep_DDMR_5Methods/Dynamics of DDMR/V(q)bar x thd (2x1)/V(q,qd)bar (3x1) ==
  phid : Inport
  Constant1 : Constant  Value=0
  Constant2 : Constant  Value=0
  Convert 1-D to 2-D : dspsigattribs/Convert 1-D to 2-D  M=2  N=2  frameBasedOut=off
  Fcn2 : Fcn  Expr=-(r^2)/2*b*mc*d*u
  Fcn3 : Fcn  Expr=(r^2)/2*b*mc*d*u
  Mux : Mux
  V(q,qd)bar : Outport
  wires:
  Convert 1-D to 2-D/1 -> V(q,qd)bar/1
  Mux/1 -> Convert 1-D to 2-D/1
  Constant2/1 -> Mux/1
  Fcn2/1 -> Mux/2
  Fcn3/1 -> Mux/3
  Constant1/1 -> Mux/4
  phid/1 -> Fcn2/1, Fcn3/1

== system ep_DDMR_5Methods/Dynamics of DDMR/direct kinematics/S(q) matrix (3x2)1 ==
  phi : Inport
  Constant1 : Constant  Value=r/(2*b)
  Constant2 : Constant  Value=-r/(2*b)
  Convert 1-D to 2-D : dspsigattribs/Convert 1-D to 2-D  M=3  N=2  frameBasedOut=off
  Fcn : Fcn  Expr=r/2*cos(u(3))+d*r/(2*b)*sin(u(3))
  Fcn1 : Fcn  Expr=r/2*sin(u(3))-d*r/(2*b)*cos(u(3))
  Fcn2 : Fcn  Expr=r/2*cos(u(3))-d*r/(2*b)*sin(u(3))
  Fcn3 : Fcn  Expr=r/2*sin(u(3))+d*r/(2*b)*cos(u(3))
  Mux : Mux  Inputs=6
  S(q) : Outport
  wires:
  Mux/1 -> Convert 1-D to 2-D/1
  Convert 1-D to 2-D/1 -> S(q)/1
  phi/1 -> Fcn3/1, Fcn2/1, Fcn/1, Fcn1/1
  Fcn/1 -> Mux/1
  Fcn1/1 -> Mux/2
  Constant2/1 -> Mux/3
  Fcn2/1 -> Mux/4
  Fcn3/1 -> Mux/5
  Constant1/1 -> Mux/6
